simulink model "sistema_LTI_equivalente"  (R2023b)
settings: Solver=VariableStepAuto  StartTime=0.0  StopTime=10.0  RelTol=1e-3
values from neighbouring files (symbols this model uses):
  b_eq = 2.1944e-5    (= 2.1944e-05)    [diagrama_polos_y_ceros_LTI.m]    (also in main.m = 2.19444444444e-05; parametros.m = 2.19444444444e-05)
  C_ts = 0.818    [parametros.m]
  J_eq = 1.9785e-5    (= 1.9785e-05)    [diagrama_polos_y_ceros_LTI.m]    (also in main.m = 1.97847222222e-05; parametros.m = 1.97847222222e-05)
  L_q = 5.8e-3    (= 0.0058)    [diagrama_polos_y_ceros_LTI.m]    (also in main.m = 5.8; parametros.m; variacion_de_parametros.m)
  lambda_m = 0.016    [main.m]    (also in parametros.m)
  P_p = 3    [diagrama_polos_y_ceros_LTI.m]    (also in main.m; parametros.m; variacion_de_parametros.m)
  R_sref = 1.02    [parametros.m]
  R_tsamb = 146.7    [parametros.m]
settings Model: Creator=nicol  LastModifiedBy=nicol

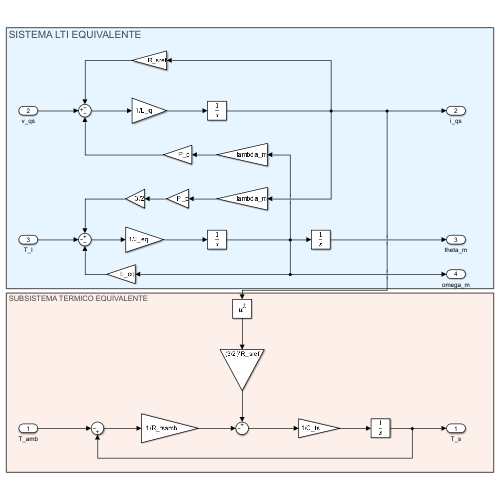
[thumbnail: Simulink's stored preview of the top-level diagram]
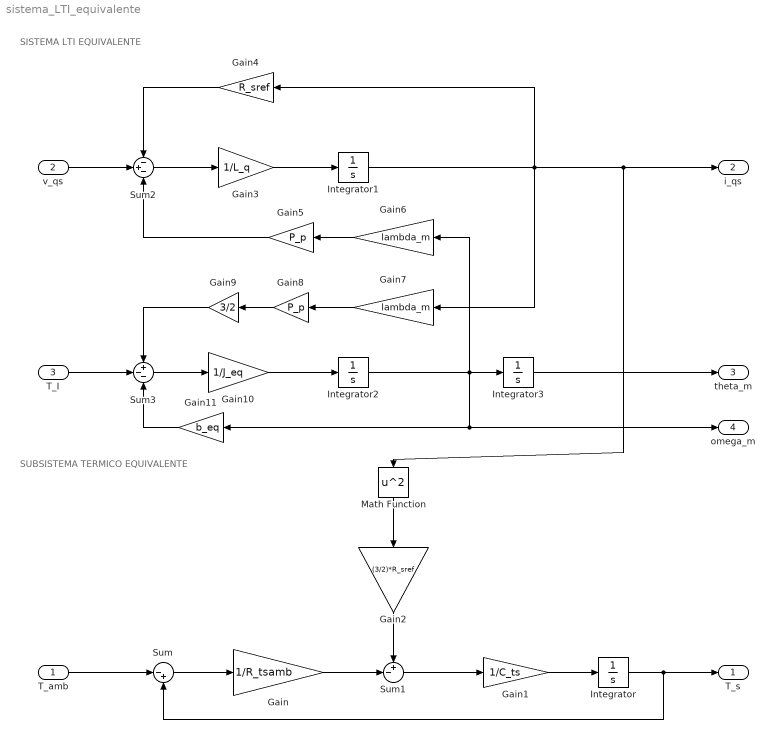
== system sistema_LTI_equivalente ==
  note: SUBSISTEMA TERMICO EQUIVALENTE
  note: SISTEMA LTI EQUIVALENTE
  T_amb : Inport
  v_qs : Inport  Port=2
  T_I : Inport  Port=3
  Gain : Gain  Gain=1/R_tsamb
  Gain1 : Gain  Gain=1/C_ts
  Gain10 : Gain  Gain=1/J_eq
  Gain11 : Gain  Gain=b_eq
  Gain2 : Gain  Gain=(3/2)*R_sref
  Gain3 : Gain  Gain=1/L_q
  Gain4 : Gain  Gain=R_sref
  Gain5 : Gain  Gain=P_p
  Gain6 : Gain  Gain=lambda_m
  Gain7 : Gain  Gain=lambda_m
  Gain8 : Gain  Gain=P_p
  Gain9 : Gain  Gain=3/2
  Integrator{,1..3} (4 alike) : Integrator
  Math Function : Math  Operator=square
  Sum : Sum  Inputs=|-+
  Sum1 : Sum  Inputs=+-|
  Sum2 : Sum  Inputs=-+-
  Sum3 : Sum  Inputs=+--
  T_s : Outport
  i_qs : Outport  Port=2
  theta_m : Outport  Port=3
  omega_m : Outport  Port=4
  wires:
  Gain1/1 -> Integrator/1
  T_amb/1 -> Sum/1
  Sum/1 -> Gain/1
  Gain/1 -> Sum1/2
  Sum1/1 -> Gain1/1
  Gain2/1 -> Sum1/1
  Integrator/1 -> Sum/2, T_s/1
  Math Function/1 -> Gain2/1
  T_I/1 -> Sum3/2
  Sum3/1 -> Gain10/1
  Gain10/1 -> Integrator2/1
  Integrator2/1 -> Gain6/1, omega_m/1, Gain11/1, Integrator3/1
  Integrator3/1 -> theta_m/1
  Gain11/1 -> Sum3/3
  Gain9/1 -> Sum3/1
  Gain8/1 -> Gain9/1
  Gain7/1 -> Gain8/1
  Gain6/1 -> Gain5/1
  Gain5/1 -> Sum2/3
  v_qs/1 -> Sum2/2
  Gain4/1 -> Sum2/1
  Sum2/1 -> Gain3/1
  Gain3/1 -> Integrator1/1
  Integrator1/1 -> Gain4/1, Gain7/1, i_qs/1, Math Function/1
